simulink model "inicjalizacja"  (R2019b)
settings: Solver=FixedStepAuto  StartTime=0.0  StopTime=inf  FixedStep=0.01  RelTol=1e-3  EnableMultiTasking=on
undefined symbols (not defined in the file or in its folder): magnitude
libraries: simulink x3, embdlinuxlib x2, dspswit3 x2, raspberrypilib x1
settings Model: SimulationMode=external  Creator=damia  LastModifiedBy=damia
settings SolverCC: PositivePriorityOrder=on
settings OptimizationCC: EnhancedBackFolding=on  PassReuseOutputArgsAs=Individual arguments  ZeroExternalMemoryAtStartup=off  ZeroInternalMemoryAtStartup=off  MaxStackSize=64  OptimizeBlockOrder=speed  DifferentSizesBufferReuse=on  OptimizationCustomize=off  EfficientTunableParamExpr=on
settings DebuggingCC: ParameterTunabilityLossMsg=error
settings HardwareCC: ProdBitPerPointer=32  ProdBitPerSizeT=32  ProdBitPerPtrDiffT=32  ProdLargestAtomicInteger=Long  ProdLargestAtomicFloat=Double  ProdWordSize=32  ProdLongLongMode=on  ProdHWDeviceType=ARM Compatible->ARM Cortex  UseEmbeddedCoderFeatures=off  UseSimulinkCoderFeatures=off
settings RTWCC: SystemTargetFile=ert.tlc  HardwareBoard=Raspberry Pi  TLCOptions="-aInlineSetEventsForThisBaseRateFcn=TLC_FALSE -aSuppressMultiTaskScheduler=TLC_FALSE  -aRateBasedStepFcn=0"  TemplateMakefile=ert_default_tmf  RTWVerbose=off  Toolchain=GNU GCC Raspberry Pi  BuildConfiguration=Faster Runs  IncludeHyperlinkInReport=on
settings CodeAppCC: ForceParamTrailComments=on  OperatorAnnotations=on  SimulinkDataObjDesc=on  SFDataObjDesc=on  MangleLength=10  InsertBlockDesc=on
settings ERTTargetCC: SupportNonInlinedSFcns=on  SupportVariableSizeSignals=on  ExtMode=on  ExtModeTransport=2  ExtModeStaticAlloc=on  ExtModeMexFile=ext_xcp  ExtModeMexArgs='192.168.1.10' 0 17725  ExtModeIntrfLevel=Level2 - Open  ERTSrcFileBannerTemplate=codertarget_code_template.cgt  ERTHdrFileBannerTemplate=codertarget_code_template.cgt  ERTDataSrcFileTemplate=codertarget_code_template.cgt  ERTDataHdrFileTemplate=codertarget_code_template.cgt

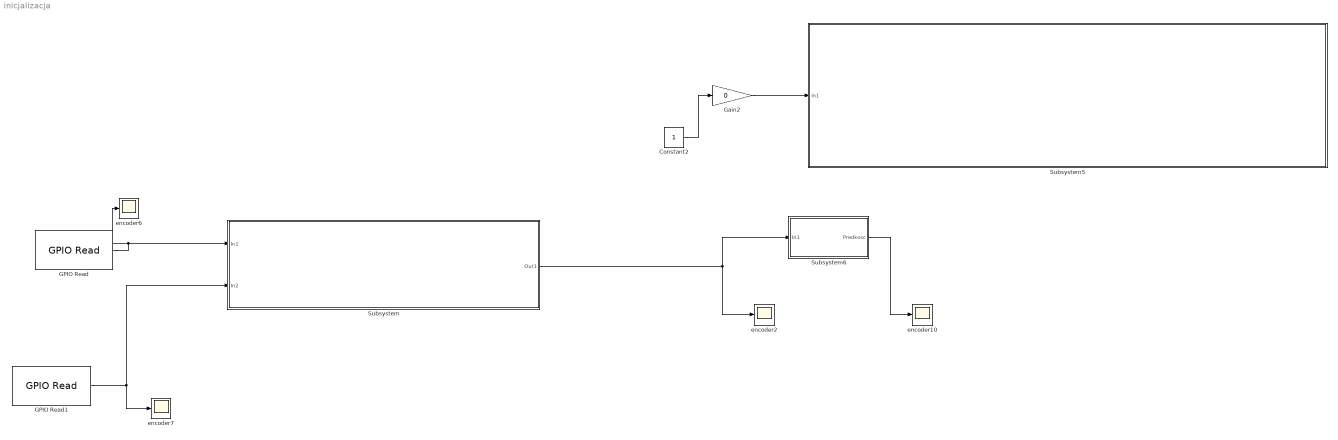
== system inicjalizacja ==
  Constant2 : Constant
  GPIO Read : embdlinuxlib/GPIO Read  board=Pi 3 Model B  gpio=14  internalResistor=Off  sampleTime=.01  direction=Input  blockPlatform=Raspberry Pi
      settings: SourceProductName=Simulink Support Package for Raspberry Pi Hardware  SourceProductBaseCode=RASPPI
  GPIO Read1 : embdlinuxlib/GPIO Read  board=Pi 3 Model B  gpio=18  internalResistor=Off  sampleTime=.01  direction=Input  blockPlatform=Raspberry Pi
      settings: SourceProductName=Simulink Support Package for Raspberry Pi Hardware  SourceProductBaseCode=RASPPI
  Gain2 : Gain  Gain=0
  Subsystem : Subsystem
  Subsystem5 : Subsystem
  Subsystem6 : Subsystem
  encoder{2,6..7,10} (4 alike) : Scope
  wires:
  Gain2/1 -> Subsystem5/1(In1)
  Subsystem/1(Out1) -> Subsystem6/1(In1), encoder2/1
  GPIO Read/1 -> encoder6/1, Subsystem/1(In1)
  GPIO Read1/1 -> Subsystem/2(In2), encoder7/1
  Constant2/1 -> Gain2/1
  Subsystem6/1(Predkosc) -> encoder10/1

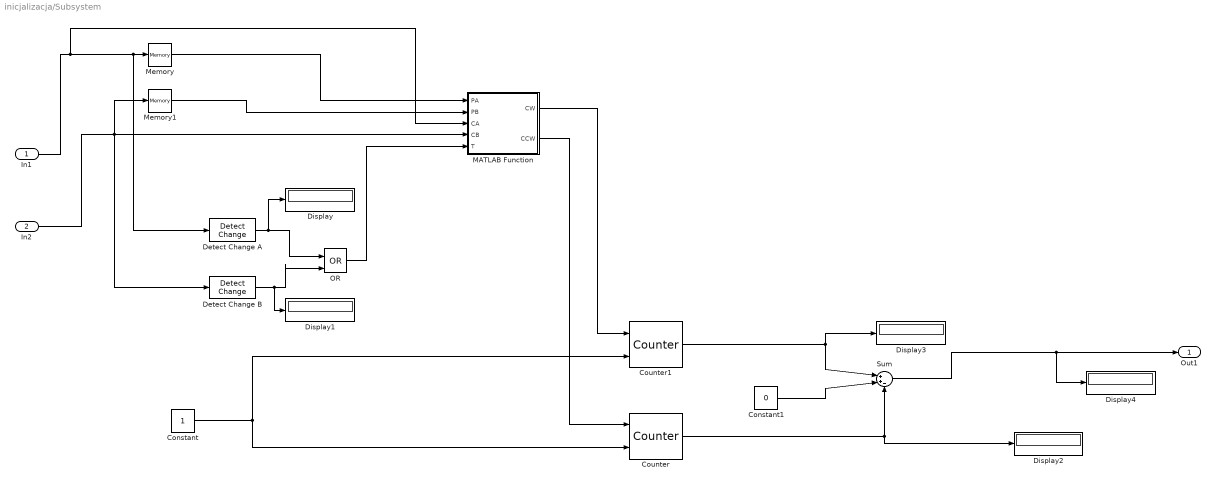
== system inicjalizacja/Subsystem ==
  In1 : Inport
  In2 : Inport  Port=2
  Constant : Constant
  Constant1 : Constant  Value=0
  Counter : dspswit3/Counter  Direction=Up  CountEvent=Rising edge  CounterSize=User defined  MaxCount=1024  InitialCount=0  Output=Count  HitValue=0  ResetInput=on  SamplesPerFrame=1  Ts=1  CntDtype=double  HitDtype=Logical
  Counter1 : dspswit3/Counter  Direction=Up  CountEvent=Rising edge  CounterSize=User defined  MaxCount=1024  InitialCount=0  Output=Count  HitValue=0  ResetInput=on  SamplesPerFrame=1  Ts=1  CntDtype=double  HitDtype=Logical
  Detect Change A : simulink/Logic and Bit Operations/Detect Change  vinit=0  OutDataTypeStr=boolean
  Detect Change B : simulink/Logic and Bit Operations/Detect Change  vinit=0  OutDataTypeStr=boolean
  Display{,1..4} (5 alike) : Display
  MATLAB Function : MATLAB Function  TreatAsAtomicUnit=on
  Memory : Memory
  Memory1 : Memory
  OR : Logic  Operator=OR  IconShape=distinctive  AllPortsSameDT=off  OutDataTypeStr=boolean
  Sum : Sum  Inputs=|++-
  Out1 : Outport
  wires:
  In1/1 -> MATLAB Function/3(CA), Detect Change A/1, Memory/1
  In2/1 -> MATLAB Function/4(CB), Detect Change B/1, Memory1/1
  Detect Change A/1 -> Display/1, OR/1
  Detect Change B/1 -> Display1/1, OR/2
  OR/1 -> MATLAB Function/5(T)
  Memory/1 -> MATLAB Function/1(PA)
  Memory1/1 -> MATLAB Function/2(PB)
  MATLAB Function/2(CCW) -> Counter/1
  MATLAB Function/1(CW) -> Counter1/1
  Constant/1 -> Counter1/2, Counter/2
  Constant1/1 -> Sum/2
  Counter/1 -> Display2/1, Sum/3
  Counter1/1 -> Sum/1, Display3/1
  Sum/1 -> Display4/1, Out1/1

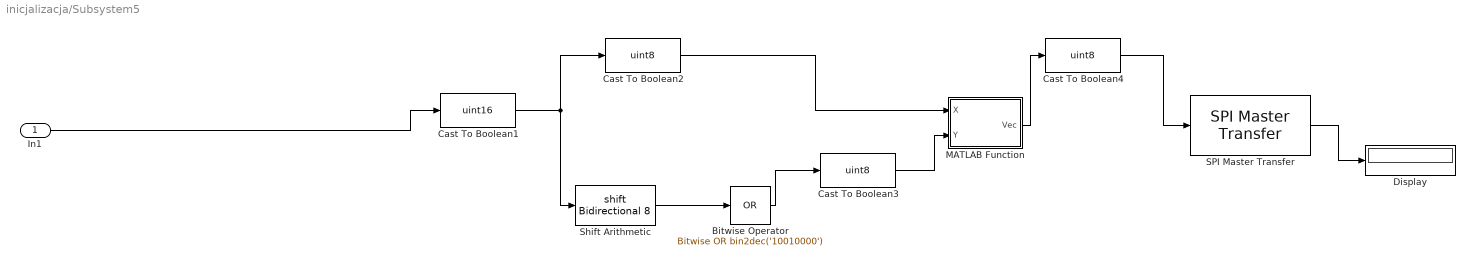
== system inicjalizacja/Subsystem5 ==
  In1 : Inport
  Bitwise Operator : simulink/Logic and Bit Operations/Bitwise Operator  logicop=OR  UseBitMask=on  BitMask=bin2dec('10010000')  BitMaskRealWorld=Real World Value
  Cast To Boolean1 : DataTypeConversion  OutDataTypeStr=uint16
  Cast To Boolean2 : DataTypeConversion  OutDataTypeStr=uint8
  Cast To Boolean3 : DataTypeConversion  OutDataTypeStr=uint8
  Cast To Boolean4 : DataTypeConversion  OutDataTypeStr=uint8
  Display : Display
  MATLAB Function : MATLAB Function  TreatAsAtomicUnit=on
  SPI Master Transfer : raspberrypilib/SPI Master Transfer  Priority=1  BoardProperty=Pi 3 Model B  SPIModule=uint32(0)  Mode=Master  BusSpeed=1000000  Pin=SPI0_CE0  FirstBitToTransfer=Most significant bit (MSB)  ClockMode=0  BlockFunction=Transfer  RegisterAddress=0  OutputDataType=int8  OutputDataLength=1
      settings: SourceProductName=Simulink Support Package for Raspberry Pi Hardware  SourceProductBaseCode=RASPPI
  Shift Arithmetic : ArithShift  BitShiftNumber=8
  wires:
  Bitwise Operator/1 -> Cast To Boolean3/1
  Cast To Boolean3/1 -> MATLAB Function/2(Y)
  Cast To Boolean4/1 -> SPI Master Transfer/1
  Shift Arithmetic/1 -> Bitwise Operator/1
  In1/1 -> Cast To Boolean1/1
  SPI Master Transfer/1 -> Display/1
  Cast To Boolean1/1 -> Cast To Boolean2/1, Shift Arithmetic/1
  MATLAB Function/1(Vec) -> Cast To Boolean4/1
  Cast To Boolean2/1 -> MATLAB Function/1(X)

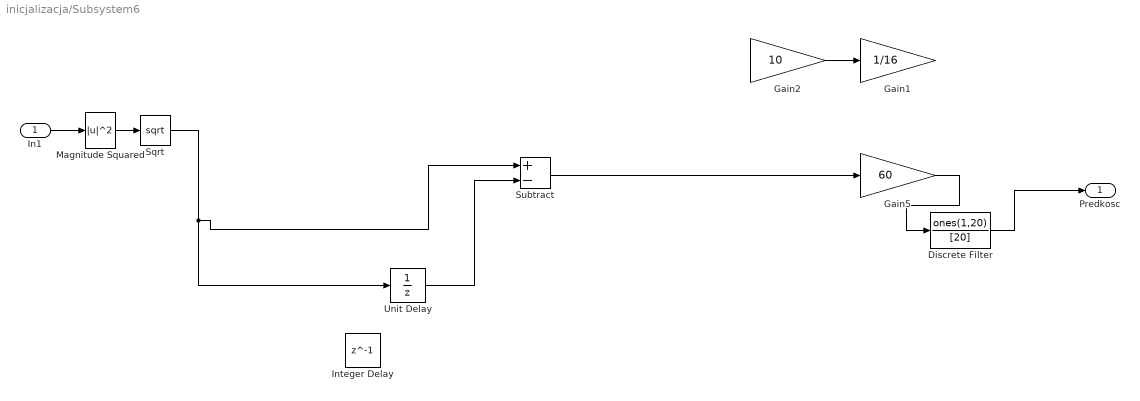
== system inicjalizacja/Subsystem6 ==
  In1 : Inport
  Discrete Filter : DiscreteFilter  Numerator=ones(1,20)  Denominator=[20]
  Gain1 : Gain  Gain=1/16  ParamDataTypeStr=double  OutDataTypeStr=int16  RndMeth=Round
  Gain2 : Gain  Gain=10  ParamDataTypeStr=double  OutDataTypeStr=int16  RndMeth=Round
  Gain5 : Gain  Gain=60  ParamDataTypeStr=double  OutDataTypeStr=int16  RndMeth=Round
  Integer Delay : Delay  DelayLength=1
  Magnitude Squared : Math  Operator=magnitude^2  SignedPower=off  SaturateOnIntegerOverflow=on
  Sqrt : Sqrt  IntermediateResultsDataTypeStr=double  SaturateOnIntegerOverflow=on
  Subtract : Sum  Inputs=+-  AccumDataTypeStr=int16  OutDataTypeStr=uint16  RndMeth=Round
  Unit Delay : UnitDelay  SampleTime=-1  HasFrameUpgradeWarning=on
  Predkosc : Outport
  wires:
  Gain2/1 -> Gain1/1
  Discrete Filter/1 -> Predkosc/1
  Unit Delay/1 -> Subtract/2
  In1/1 -> Magnitude Squared/1
  Gain5/1 -> Discrete Filter/1
  Subtract/1 -> Gain5/1
  Magnitude Squared/1 -> Sqrt/1
  Sqrt/1 -> Unit Delay/1, Subtract/1

== matlab function inicjalizacja/Subsystem5/MATLAB Function ==
  data: X input; Vec output; Y input
function Vec = Vector(X, Y)

% myPI = raspi();
Vec = [Y X];
% mySPI = spidev(myPI,'CE0');
% out = writeRead(mySPI,[Vec]);

== matlab function inicjalizacja/Subsystem/MATLAB Function ==
  data: PA input; CW output; PB input; CCW output; CA input; CB input; T input
function [CW,CCW] = encoder(PA,PB,CA,CB,T)

% persistent counter;
% if isempty(counter)
% counter = 0;
% end
% persistent aLastState;
% if isempty(aLastState)
% aLastState = a;
% end
% % 
% % out = aLastState
% % while(1)
%     aState = a;
%     bState = b;
%     if(aState ~= aLastState)
%         bstate = b;
%     end
%     if(bState ~=aState)
%         counter = counter+1;
%     else
%         counter = counter - 1;
%     end
%      out = counter;
%     aLastState = aState;
% end

CW = NaN; CCW = NaN;
if(T==1)
    if PA == 0
        if PB == 0
        if CA == 0 && CB == 1  %0001
            CW = 1;
            CCW = 0;
        elseif CA == 1 && CB == 0 %0010
            CW = 0;
            CCW = 1;
        end
    elseif PB == 1
        if CA == 1 && CB == 1 %0111
            CW=1;
            CCW=0;
        elseif CA == 0 && CB == 0 %0100
            CW = 0;
            CCW = 1;
        end
    end
elseif PA == 1
    if PB == 1
        if CA == 1 && CB == 0  % 1110
            CW = 1;
            CCW = 0;
        elseif CA == 0 && CB == 1  %1101
            CW = 0;
            CCW = 1;
        end
        
    elseif PB == 0 
        if CA == 0 && CB == 0  % 1000
            CW = 1; 
            CCW = 0;
        elseif CA == 1 && CB == 1 %1011
            CW = 0; 
            CCW = 1;
        end
    end
end
end
end
